simulink model "B4_quadcopter_model_discrete"  (R2021b)
settings: Solver=VariableStepAuto  StartTime=0.0  StopTime=10  FixedStep=0.002  RelTol=1e-3
values from neighbouring files (symbols this model uses):
  coef_sim_1 = tf_des_d.Denominator{1}(2)    [A11_setup_script_pprz.m]    (also in A1_setup_script.m; A6_slow_actuator.m)
  coef_sim_2 = tf_des_d.Numerator{1}(2)    [A11_setup_script_pprz.m]    (also in A1_setup_script.m; A6_slow_actuator.m)
  doublet_mag = - 0.15    (= -0.15)    [A11_setup_script_pprz.m]    (also in A1_setup_script.m)
  doublet_time = 6    [A11_setup_script_pprz.m]    (also in A1_setup_script.m)
  f_8 = 1    [A11_setup_script_pprz.m]    (also in A1_setup_script.m)
  FILT_CUTOFF = 2*pi*5    (= 31.4159265359)    [A11_setup_script_pprz.m]    (also in A1_setup_script.m)
  FILTER = 1    [A11_setup_script_pprz.m]    (also in A1_setup_script.m)
  G1 = inv(I)*G1_r    [A10_simple_plant.m]    (also in A11_setup_script_pprz.m = G1/scale; A1_setup_script.m = [G1;G1_T])
  G1_simple = inv(I)*G1_r_simple    [A1_setup_script.m]
  G2 = G2/scale    [A11_setup_script_pprz.m]    (also in A1_setup_script.m = (1/sampling_time)*inv(I)*(G2_r))
  h_plate = 0.3    [A11_setup_script_pprz.m]    (also in A1_setup_script.m = 0.16)
  I = eye(3,3)    [A10_simple_plant.m]    (also in A11_setup_script_pprz.m; A1_setup_script.m; A2_B_matrix_generation_symbolic.m = [Ixx 0 0; A3_B_matrix_generation_symbolic_cascaded.m = [Ixx 0 0)
  Iyy = 0.0008    [A11_setup_script_pprz.m]    (also in A1_setup_script.m = 0.0015)
  Izz = 0.000498    [A11_setup_script_pprz.m]    (also in A1_setup_script.m = 0.00015)
  K = 7    [A11_setup_script_pprz.m]    (also in A1_setup_script.m = 10)
  K_act = 50    [A10_simple_plant.m]    (also in A11_setup_script_pprz.m = 20; A1_setup_script.m = 20)
  K_act_outer = diag([K K K_act])    [A1_setup_script.m]
  K_d = 15    [A11_setup_script_pprz.m]    (also in A1_setup_script.m = 25)
  K_dd = K_act    (= 20)    [A11_setup_script_pprz.m]    (also in A1_setup_script.m)
  K_dyn = K    (= 10)    [A1_setup_script.m]
  K_ec = 50    [A11_setup_script_pprz.m]    (also in A1_setup_script.m = 251)
  K_ec_d = 13    [A11_setup_script_pprz.m]    (also in A1_setup_script.m = 25)
  K_ec_d_u = 1.5    [A11_setup_script_pprz.m]    (also in A1_setup_script.m = 5)
  K_ec_d_v = 1.5    [A11_setup_script_pprz.m]    (also in A1_setup_script.m = 5)
  K_ec_d_w = 1.5    [A11_setup_script_pprz.m]    (also in A1_setup_script.m = 5)
  K_ec_dd = 9    [A11_setup_script_pprz.m]    (also in A1_setup_script.m = 45)
  K_ec_i = 0    [A11_setup_script_pprz.m]    (also in A1_setup_script.m = 380)
  K_ec_u = 1.5    [A11_setup_script_pprz.m]    (also in A1_setup_script.m = 5)
  K_ec_v = 1.5    [A11_setup_script_pprz.m]    (also in A1_setup_script.m = 5)
  K_ec_w = 1.5    [A11_setup_script_pprz.m]    (also in A1_setup_script.m = 5)
  K_t = 0.0005    [A10_simple_plant.m]    (also in A11_setup_script_pprz.m = 6.557e-08; A1_setup_script.m = 6.557e-08)
  K_u = 1.0    (= 1)    [A11_setup_script_pprz.m]    (also in A1_setup_script.m = 1.5)
  K_u_d = 2.5    [A11_setup_script_pprz.m]    (also in A1_setup_script.m = 7)
  K_u_dd = K    (= 10)    [A1_setup_script.m]
  K_v = 1.0    (= 1)    [A11_setup_script_pprz.m]    (also in A1_setup_script.m = 1.5)
  K_v_d = 2.5    [A11_setup_script_pprz.m]    (also in A1_setup_script.m = 7)
  K_v_dd = K    (= 10)    [A1_setup_script.m]
  K_w = 1.0    (= 1)    [A11_setup_script_pprz.m]    (also in A1_setup_script.m = 4.5)
  K_w_d = 2.5    [A11_setup_script_pprz.m]    (also in A1_setup_script.m = 7)
  K_w_dd = K    (= 10)    [A1_setup_script.m]
  l_plate = 0.1    [A11_setup_script_pprz.m]    (also in A1_setup_script.m = 0.11)
  m = 0.4    [A10_simple_plant.m]    (also in A11_setup_script_pprz.m; A1_setup_script.m)
  NOISE = 0    [A11_setup_script_pprz.m]    (also in A1_setup_script.m)
  NOISE_ACC = 0.00005    (= 5e-05)    [A11_setup_script_pprz.m]    (also in A1_setup_script.m)
  NOISE_GYRO = 0.00005    (= 5e-05)    [A11_setup_script_pprz.m]    (also in A1_setup_script.m)
  NOISE_RPM = 200    [A11_setup_script_pprz.m]    (also in A1_setup_script.m)
  omega_act = 50    [A6_slow_actuator.m]
  omega_des = 20.00    (= 20)    [A11_setup_script_pprz.m]    (also in A1_setup_script.m; A6_slow_actuator.m = 49)
  sampling_time = 1/frequency    (= 0.002)    [A11_setup_script_pprz.m]    (also in A12_sim_multi_run.m; A1_setup_script.m; A6_slow_actuator.m)
  scale_8 = 1.6    [A11_setup_script_pprz.m]    (also in A1_setup_script.m)
  start_8 = 2    [A11_setup_script_pprz.m]    (also in A1_setup_script.m)
  start_time = 2    [A11_setup_script_pprz.m]    (also in A1_setup_script.m = 1)
  t_8 = 10    [A11_setup_script_pprz.m]    (also in A1_setup_script.m)
  w_plate = 0.3    [A11_setup_script_pprz.m]    (also in A1_setup_script.m = 0.36)
undefined symbols (not defined in the file or in its folder): DiscIntNeverNeededParam, K_ec_d_p, K_ec_d_q, K_ec_d_r, K_ec_dd_p, K_ec_dd_q, K_ec_dd_r, K_ec_i_u, K_ec_i_v, K_ec_i_w, K_ec_p, K_ec_q, K_ec_r, K_p, K_p_d, K_p_dd, K_q, K_q_d, K_q_dd, K_r, K_r_d, K_r_dd
libraries: simulink x44, cstblocks x37, dspinverses x26, dspmathops x9, dspstat3 x9, aerolibutil x9, sharedutil x3, aerolibanim x1
(part 2 of 13)

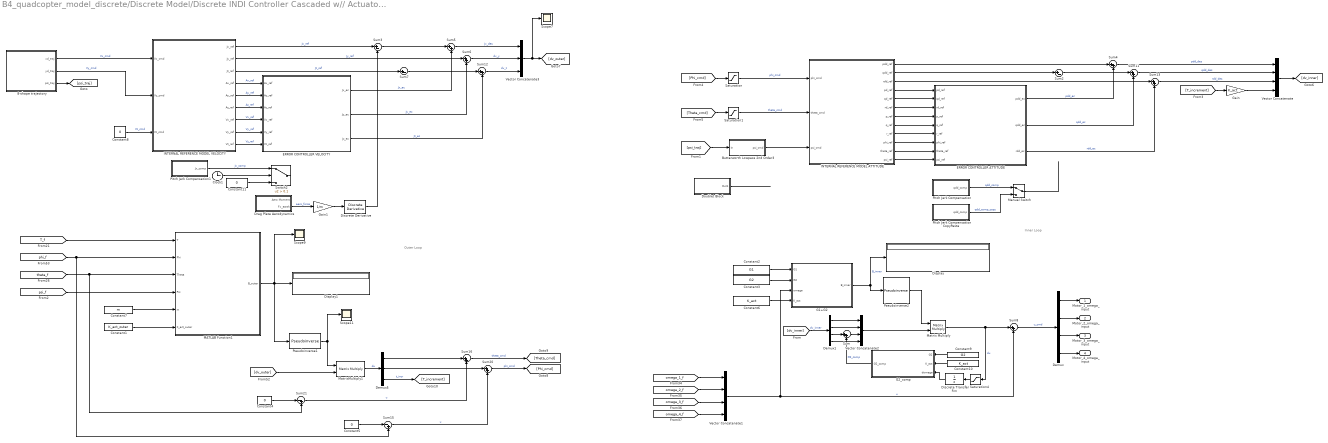
== system B4_quadcopter_model_discrete/Discrete Model/Discrete INDI Controller Cascaded w// Actuator Compensation Double ==
  note: Outer Loop
  note: Inner Loop
  8-shape trajectory : Subsystem
  Butterworth Lowpass 2nd Order3 : Subsystem
  Clock1 : Clock
      settings: Decimation=100
  Constant1 : Constant  Value=K_act_outer  SampleTime=sampling_time
  Constant10 : Constant  Value=K_act  SampleTime=sampling_time
  Constant11 : Constant  Value=0
  Constant2 : Constant  Value=G1  SampleTime=sampling_time
  Constant3 : Constant  Value=G2  SampleTime=sampling_time
  Constant4 : Constant  Value=0
  Constant5 : Constant  Value=0
  Constant6 : Constant  Value=K_act  SampleTime=sampling_time
  Constant7 : Constant  Value=m  SampleTime=sampling_time
  Constant8 : Constant  Value=0  SampleTime=sampling_time
  Constant9 : Constant  Value=G2  SampleTime=sampling_time
  Demux : Demux
  Demux1 : Demux
  Demux5 : Demux  Outputs=3
  Discrete Transfer Fcn : DiscreteTransferFcn  Denominator=[1 0]
  Discrete Derivative : simulink/Discrete/Discrete Derivative  gainval=1.0  ICPrevScaledInput=0.0  OutMin=[]  OutMax=[]  OutDataType=fixdt(1, 16)  OutScaling=2^-10  DoSatur=off
  Display : Display
  Display1 : Display
  Doublet Block : Subsystem
  Drag Plate Aerodynamics : Subsystem
  ERROR CONTROLLER ATTITUDE : Subsystem
  ERROR CONTROLLER VELOCITY : Subsystem
  G1+G2 : MATLAB Function  TreatAsAtomicUnit=on
  G2_comp : MATLAB Function  TreatAsAtomicUnit=on
  Gain : Gain  Gain=K_act
  Gain1 : Gain  Gain=1/m
  INTERNAL REFERENCE MODEL ATTITUDE : Subsystem
  INTERNAL REFERENCE MODEL VELOCITY : Subsystem
  MATLAB Function1 : MATLAB Function  TreatAsAtomicUnit=on
  Manual Switch : ManualSwitch
  Matrix Multiply : Product  Multiplication=Matrix(*)
  MatrixMultiply1 : Product  Multiplication=Matrix(*)
  Pitch Jerk Compensation : Subsystem
  Pitch Jerk Compensation CopyPaste : Subsystem
  Pitch Jerk Compensation1 : Subsystem
  Pseudoinverse1 : dspinverses/Pseudoinverse  wanterr=off  SimulateUsing=Interpreted execution
      settings: SourceProductBaseCode=DS
  Pseudoinverse2 : dspinverses/Pseudoinverse  wanterr=off  SimulateUsing=Interpreted execution
      settings: SourceProductBaseCode=DS
  Saturation : Saturate
  Saturation1 : Saturate
  Saturation4 : Saturate  UpperLimit=12000  LowerLimit=10
  Scope11 : Scope
  Scope7 : Scope
  Scope9 : Scope
  Sum{,4..6,8,11..13,16,20} (10 alike) : Sum  Inputs=|++
  Sum15 : Sum  Inputs=|-+
  Sum2 : Sum  Inputs=|+-
  Sum21 : Sum  Inputs=|-+
  Sum3 : Sum  Inputs=|+-
  Sum7 : Sum  Inputs=|+-
  Switch2 : Switch  Criteria=u2 > Threshold  Threshold=0.1
  Vector Concatenate : Concatenate  NumInputs=4
  Vector Concatenate1 : Concatenate  NumInputs=4
  Vector Concatenate2 : Concatenate  NumInputs=4
  Vector Concatenate3 : Concatenate  NumInputs=3
  Motor_1_omega_input : Outport
  Motor_2_omega_input : Outport  Port=2
  Motor_3_omega_input : Outport  Port=3
  Motor_4_omega_input : Outport  Port=4
  wires:
  Constant4/1 -> Sum21/1
  Sum16/1 -> [Theta_cmd]  "theta_cmd"
  Sum12/1 -> Vector Concatenate3/3  "dv_z"
  INTERNAL REFERENCE MODEL VELOCITY/2(Jy_ref) -> Sum6/1  "Jy_ref"
  Sum21/1 -> Sum16/2  "u"
  ERROR CONTROLLER VELOCITY/2(Jy_ec) -> Sum6/2  "Jy_ec"
  8-shape trajectory/1(xd_traj) -> INTERNAL REFERENCE MODEL VELOCITY/1(Vx_cmd)  "Vx_cmd"
  Sum6/1 -> Vector Concatenate3/2  "dv_y"
  ERROR CONTROLLER VELOCITY/1(Jx_ec) -> Sum5/2  "Jx_ec"
  Sum5/1 -> Vector Concatenate3/1  "Jx_des"
  ERROR CONTROLLER VELOCITY/3(Jz_ec) -> Sum12/2  "Jz_ec"
  Constant8/1 -> INTERNAL REFERENCE MODEL VELOCITY/3(Vz_cmd)  "Vz_cmd"
  Pseudoinverse1/1 -> Scope11/1, MatrixMultiply1/1
  Sum15/1 -> Sum20/2  "u"
  Vector Concatenate3/1 -> Scope7/1, [dv_outer]
  INTERNAL REFERENCE MODEL VELOCITY/1(Jx_ref) -> Sum3/1  "Jx_ref"
  INTERNAL REFERENCE MODEL VELOCITY/3(Jz_ref) -> Sum7/1  "Jz_ref"
  Sum20/1 -> [Phi_cmd]  "phi_cmd"
  [T_f] -> MATLAB Function1/1(T)
  Constant7/1 -> MATLAB Function1/5(m)
  Constant5/1 -> Sum15/1
  [dv_outer] -> MatrixMultiply1/2
  Demux5/1 -> Sum16/1
  MATLAB Function1/1(B_outer) -> Pseudoinverse1/1, Display1/1, Scope9/1
  Demux5/3 -> [T_increment]  "t_incr"
  MatrixMultiply1/1 -> Demux5/1  "du"
  Demux5/2 -> Sum20/1
  8-shape trajectory/2(yd_traj) -> INTERNAL REFERENCE MODEL VELOCITY/2(Vy_cmd)  "Vy_cmd"
  [theta_f] -> Sum21/2, MATLAB Function1/3(Theta)
  [phi_f] -> Sum15/2, MATLAB Function1/2(Phi)
  8-shape trajectory/3(psi_traj) -> [psi_traj]
  INTERNAL REFERENCE MODEL VELOCITY/4(Ax_ref) -> ERROR CONTROLLER VELOCITY/1(Ax_ref)  "Ax_ref"
  INTERNAL REFERENCE MODEL VELOCITY/5(Ay_ref) -> ERROR CONTROLLER VELOCITY/2(Ay_ref)  "Ay_ref"
  INTERNAL REFERENCE MODEL VELOCITY/6(Az_ref) -> ERROR CONTROLLER VELOCITY/3(Az_ref)  "Az_ref"
  INTERNAL REFERENCE MODEL VELOCITY/7(Vx_ref) -> ERROR CONTROLLER VELOCITY/4(Vx_ref)  "Vx_ref"
  INTERNAL REFERENCE MODEL VELOCITY/8(Vy_ref) -> ERROR CONTROLLER VELOCITY/5(Vy_ref)  "Vy_ref"
  INTERNAL REFERENCE MODEL VELOCITY/9(Vz_ref) -> ERROR CONTROLLER VELOCITY/6(Vz_ref)  "Vz_ref"
  Sum3/1 -> Sum5/1
  Sum7/1 -> Sum12/1
  Constant1/1 -> MATLAB Function1/6(K_act_outer)
  [psi_f] -> MATLAB Function1/4(Psi)
  INTERNAL REFERENCE MODEL ATTITUDE/12(psi_ref) -> ERROR CONTROLLER ATTITUDE/9(psi_ref)
  Demux1/1 -> Vector Concatenate2/1
  ERROR CONTROLLER ATTITUDE/2(qdd_ec) -> Sum11/2  "qdd_ec"
  Sum4/1 -> Vector Concatenate/1  "pdd_des"
  [dv_inner] -> Demux1/1  "dv_inner"
  Demux1/4 -> Vector Concatenate2/4
  INTERNAL REFERENCE MODEL ATTITUDE/3(rdd_ref) -> Sum13/1
  Sum2/1 -> Sum11/1
  INTERNAL REFERENCE MODEL ATTITUDE/9(r_ref) -> ERROR CONTROLLER ATTITUDE/6(r_ref)
  [omega_2_f] -> Vector Concatenate1/2
  Sum11/1 -> Vector Concatenate/2  "qdd_des"
  INTERNAL REFERENCE MODEL ATTITUDE/10(phi_ref) -> ERROR CONTROLLER ATTITUDE/7(phi_ref)
  Demux1/2 -> Vector Concatenate2/2
  G2_comp/1(G2_comp) -> Sum/2  "G2_comp"
  Saturation1/1 -> INTERNAL REFERENCE MODEL ATTITUDE/2(theta_cmd)  "theta_cmd"
  [Theta_cmd] -> Saturation1/1
  Demux/3 -> Motor_3_omega_input/1
  INTERNAL REFERENCE MODEL ATTITUDE/4(pd_ref) -> ERROR CONTROLLER ATTITUDE/1(pd_ref)
  Saturation/1 -> INTERNAL REFERENCE MODEL ATTITUDE/1(phi_cmd)  "phi_cmd"
  Doublet Block/1(Out1) -> ?
  INTERNAL REFERENCE MODEL ATTITUDE/7(p_ref) -> ERROR CONTROLLER ATTITUDE/4(p_ref)
  Sum/1 -> Vector Concatenate2/3
  Demux1/3 -> Sum/1
  [omega_1_f] -> Vector Concatenate1/1
  INTERNAL REFERENCE MODEL ATTITUDE/2(qdd_ref) -> Sum2/1
  INTERNAL REFERENCE MODEL ATTITUDE/11(theta_ref) -> ERROR CONTROLLER ATTITUDE/8(theta_ref)
  Constant3/1 -> G1+G2/2(G2)
  Vector Concatenate1/1 -> G1+G2/3(omega), Sum8/2  "u"
  Saturation4/1 -> Discrete Transfer Fcn/1
  Pseudoinverse2/1 -> Matrix Multiply/1
  Demux/4 -> Motor_4_omega_input/1
  Butterworth Lowpass 2nd Order3/1(psi_cmd) -> INTERNAL REFERENCE MODEL ATTITUDE/3(psi_cmd)
  Sum13/1 -> Vector Concatenate/3  "rdd_des"
  Vector Concatenate2/1 -> Matrix Multiply/2
  ERROR CONTROLLER ATTITUDE/3(rdd_ec) -> Sum13/2  "rdd_ec"
  Constant10/1 -> G2_comp/2(K_act)
  [omega_4_f] -> Vector Concatenate1/4
  ERROR CONTROLLER ATTITUDE/1(pdd_ec) -> Sum4/2  "pdd_ec"
  Discrete Transfer Fcn/1 -> G2_comp/3(domega)
  INTERNAL REFERENCE MODEL ATTITUDE/8(q_ref) -> ERROR CONTROLLER ATTITUDE/5(q_ref)
  Pitch Jerk Compensation CopyPaste/1(qdd_comp) -> Manual Switch/2  "qdd_comp_copy"
  Demux/2 -> Motor_2_omega_input/1
  Constant2/1 -> G1+G2/1(G1)
  Constant9/1 -> G2_comp/1(G2)
  INTERNAL REFERENCE MODEL ATTITUDE/1(pdd_ref) -> Sum4/1
  G1+G2/1(B_inner) -> Pseudoinverse2/1, Display/1  "B_inner"
  [T_increment] -> Gain/1
  Demux/1 -> Motor_1_omega_input/1
  [psi_traj] -> Butterworth Lowpass 2nd Order3/1(In)
  Constant6/1 -> G1+G2/4(K_act)
  INTERNAL REFERENCE MODEL ATTITUDE/6(rd_ref) -> ERROR CONTROLLER ATTITUDE/3(rd_ref)
  Manual Switch/1 -> ?
  Vector Concatenate/1 -> [dv_inner]
  Sum8/1 -> Demux/1  "u_cmd"
  [omega_3_f] -> Vector Concatenate1/3
  INTERNAL REFERENCE MODEL ATTITUDE/5(qd_ref) -> ERROR CONTROLLER ATTITUDE/2(qd_ref)
  Gain/1 -> Vector Concatenate/4
  [Phi_cmd] -> Saturation/1
  Matrix Multiply/1 -> Saturation4/1, Sum8/1  "du"
  Pitch Jerk Compensation/1(qdd_comp) -> Manual Switch/1  "qdd_comp"
  Constant11/1 -> Switch2/3
  Pitch Jerk Compensation1/1(Jx_comp) -> Switch2/1  "Jx_comp"
  Clock1/1 -> Switch2/2
  Drag Plate Aerodynamics/2(Fx_earth) -> Gain1/1  "aero_force"
  Gain1/1 -> Discrete Derivative/1
  Discrete Derivative/1 -> Sum3/2

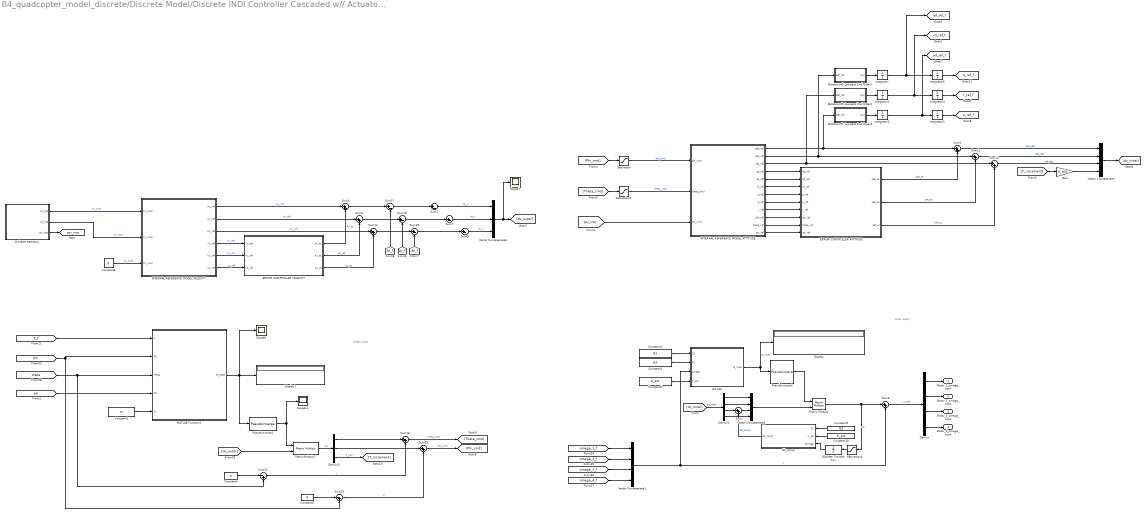
== system B4_quadcopter_model_discrete/Discrete Model/Discrete INDI Controller Cascaded w// Actuator Compensation1 ==
  note: Inner Loop
  note: Outer Loop
  8-shape trajectory : Subsystem
  Butterworth Lowpass 2nd Order1 : Subsystem
  Butterworth Lowpass 2nd Order2 : Subsystem
  Butterworth Lowpass 2nd Order3 : Subsystem
  Constant1 : Constant  Value=m  SampleTime=sampling_time
  Constant10 : Constant  Value=K_act  SampleTime=sampling_time
  Constant2 : Constant  Value=G1  SampleTime=sampling_time
  Constant3 : Constant  Value=G2  SampleTime=sampling_time
  Constant4 : Constant  Value=0
  Constant5 : Constant  Value=0
  Constant6 : Constant  Value=K_act  SampleTime=sampling_time
  Constant8 : Constant  Value=0  SampleTime=sampling_time
  Constant9 : Constant  Value=G2  SampleTime=sampling_time
  Demux : Demux
  Demux1 : Demux
  Demux5 : Demux  Outputs=3
  Discrete Transfer Fcn : DiscreteTransferFcn  Denominator=[1 0]
  Display : Display
  Display1 : Display
  ERROR CONTROLLER ATTITUDE : Subsystem
  ERROR CONTROLLER VELOCITY : Subsystem
  G1+G2 : MATLAB Function  TreatAsAtomicUnit=on
  G2_comp : MATLAB Function  TreatAsAtomicUnit=on
  Gain : Gain  Gain=K_act
  INTERNAL REFERENCE MODEL ATTITUDE : Subsystem
  INTERNAL REFERENCE MODEL VELOCITY : Subsystem
  Integrator{,1..5} (6 alike) : Integrator
  MATLAB Function1 : MATLAB Function  TreatAsAtomicUnit=on
  Matrix Multiply : Product  Multiplication=Matrix(*)
  MatrixMultiply1 : Product  Multiplication=Matrix(*)
  Pseudoinverse1 : dspinverses/Pseudoinverse  wanterr=off  SimulateUsing=Interpreted execution
      settings: SourceProductBaseCode=DS
  Pseudoinverse2 : dspinverses/Pseudoinverse  wanterr=off  SimulateUsing=Interpreted execution
      settings: SourceProductBaseCode=DS
  Saturation : Saturate
  Saturation1 : Saturate
  Saturation4 : Saturate  UpperLimit=12000  LowerLimit=10
  Scope11 : Scope
  Scope7 : Scope
  Scope9 : Scope
  Sum{,4..6,8,11..13,16,20} (10 alike) : Sum  Inputs=|++
  Sum15 : Sum  Inputs=|-+
  Sum{3,7,9,17..19} (6 alike) : Sum  Inputs=|+-
  Sum21 : Sum  Inputs=|-+
  Vector Concatenate : Concatenate  NumInputs=4
  Vector Concatenate1 : Concatenate  NumInputs=4
  Vector Concatenate2 : Concatenate  NumInputs=4
  Vector Concatenate3 : Concatenate  NumInputs=3
  Motor_1_omega_input : Outport
  Motor_2_omega_input : Outport  Port=2
  Motor_3_omega_input : Outport  Port=3
  Motor_4_omega_input : Outport  Port=4
  tag scope: p_ref_f=global, pd_ref_f=global, psi_traj=global, q_ref_f=global, qd_ref_f=global, r_ref_f=global, rd_ref_f=global
  wires:
  G1+G2/1(B_inner) -> Pseudoinverse2/1, Display/1  "B_inner"
  Vector Concatenate1/1 -> G1+G2/3(omega), Sum8/2  "u"
  Vector Concatenate/1 -> [dv_inner]
  Matrix Multiply/1 -> Saturation4/1, Sum8/1  "du"
  Demux/1 -> Motor_1_omega_input/1
  [omega_4_f] -> Vector Concatenate1/4
  [omega_2_f] -> Vector Concatenate1/2
  Demux/3 -> Motor_3_omega_input/1
  Sum8/1 -> Demux/1  "u_cmd"
  Pseudoinverse2/1 -> Matrix Multiply/1
  [omega_1_f] -> Vector Concatenate1/1
  Demux/2 -> Motor_2_omega_input/1
  Demux/4 -> Motor_4_omega_input/1
  [omega_3_f] -> Vector Concatenate1/3
  INTERNAL REFERENCE MODEL VELOCITY/5(Vy_ref) -> ERROR CONTROLLER VELOCITY/2(Vy_ref)  "Vy_ref"
  Constant4/1 -> Sum21/1
  Sum16/1 -> [Theta_cmd]  "theta_cmd"
  Sum9/1 -> Vector Concatenate3/3  "dv_z"
  INTERNAL REFERENCE MODEL VELOCITY/2(Ay_ref) -> Sum6/1  "Ay_ref"
  Sum21/1 -> Sum16/2  "u"
  INTERNAL REFERENCE MODEL VELOCITY/6(Vz_ref) -> ERROR CONTROLLER VELOCITY/3(Vz_ref)  "Vz_ref"
  INTERNAL REFERENCE MODEL VELOCITY/4(Vx_ref) -> ERROR CONTROLLER VELOCITY/1(Vx_ref)  "Vx_ref"
  ERROR CONTROLLER VELOCITY/2(Ay_ec) -> Sum6/2  "Ay_ec"
  8-shape trajectory/1(xd_traj) -> INTERNAL REFERENCE MODEL VELOCITY/1(Vx_cmd)  "Vx_cmd"
  Sum7/1 -> Vector Concatenate3/2  "dv_y"
  ERROR CONTROLLER VELOCITY/1(Ax_ec) -> Sum5/2  "Ax_ec"
  Sum3/1 -> Vector Concatenate3/1  "dv_x"
  ERROR CONTROLLER VELOCITY/3(Az_ec) -> Sum12/2  "Az_ec"
  Sum12/1 -> Sum19/1
  Constant8/1 -> INTERNAL REFERENCE MODEL VELOCITY/3(Vz_cmd)  "Vz_cmd"
  Pseudoinverse1/1 -> Scope11/1, MatrixMultiply1/1
  Sum15/1 -> Sum20/2  "u"
  Vector Concatenate3/1 -> Scope7/1, [dv_outer]
  INTERNAL REFERENCE MODEL VELOCITY/1(Ax_ref) -> Sum5/1  "Ax_ref"
  INTERNAL REFERENCE MODEL VELOCITY/3(Az_ref) -> Sum12/1  "Az_ref"
  Sum20/1 -> [Phi_cmd]  "phi_cmd"
  [T_f] -> MATLAB Function1/1(T)
  Sum6/1 -> Sum18/1
  Constant5/1 -> Sum15/1
  [dv_outer] -> MatrixMultiply1/2
  MATLAB Function1/1(B_outer) -> Scope9/1, Display1/1, Pseudoinverse1/1
  Demux5/3 -> [T_increment]  "t_incr"
  MatrixMultiply1/1 -> Demux5/1  "du"
  8-shape trajectory/2(yd_traj) -> INTERNAL REFERENCE MODEL VELOCITY/2(Vy_cmd)  "Vy_cmd"
  [T_increment] -> Gain/1
  [Ax_f] -> Sum17/2
  [Ay_f] -> Sum18/2
  [Az_f] -> Sum19/2
  [Phi_cmd] -> Saturation/1
  [theta] -> Sum21/2, MATLAB Function1/3(Theta)
  [phi] -> Sum15/2, MATLAB Function1/2(Phi)
  INTERNAL REFERENCE MODEL ATTITUDE/4(pd_ref) -> ERROR CONTROLLER ATTITUDE/1(pd_ref)
  INTERNAL REFERENCE MODEL ATTITUDE/7(p_ref) -> ERROR CONTROLLER ATTITUDE/4(p_ref)
  ERROR CONTROLLER ATTITUDE/3(rdd_ec) -> Sum13/2  "rdd_ec"
  ERROR CONTROLLER ATTITUDE/2(qdd_ec) -> Sum11/2  "qdd_ec"
  INTERNAL REFERENCE MODEL ATTITUDE/5(qd_ref) -> ERROR CONTROLLER ATTITUDE/2(qd_ref)
  INTERNAL REFERENCE MODEL ATTITUDE/11(theta_ref) -> ERROR CONTROLLER ATTITUDE/8(theta_ref)
  INTERNAL REFERENCE MODEL ATTITUDE/1(pdd_ref) -> Sum4/1, Butterworth Lowpass 2nd Order3/1(qdd_ref)
  INTERNAL REFERENCE MODEL ATTITUDE/3(rdd_ref) -> Butterworth Lowpass 2nd Order2/1(qdd_ref), Sum13/1
  INTERNAL REFERENCE MODEL ATTITUDE/8(q_ref) -> ERROR CONTROLLER ATTITUDE/5(q_ref)
  ERROR CONTROLLER ATTITUDE/1(pdd_ec) -> Sum4/2  "pdd_ec"
  INTERNAL REFERENCE MODEL ATTITUDE/6(rd_ref) -> ERROR CONTROLLER ATTITUDE/3(rd_ref)
  INTERNAL REFERENCE MODEL ATTITUDE/10(phi_ref) -> ERROR CONTROLLER ATTITUDE/7(phi_ref)
  INTERNAL REFERENCE MODEL ATTITUDE/12(psi_ref) -> ERROR CONTROLLER ATTITUDE/9(psi_ref)
  INTERNAL REFERENCE MODEL ATTITUDE/9(r_ref) -> ERROR CONTROLLER ATTITUDE/6(r_ref)
  Sum13/1 -> Vector Concatenate/3  "rdd_des"
  Sum4/1 -> Vector Concatenate/1  "pdd_des"
  Sum11/1 -> Vector Concatenate/2  "qdd_des"
  Gain/1 -> Vector Concatenate/4
  Constant3/1 -> G1+G2/2(G2)
  Constant6/1 -> G1+G2/4(K_act)
  Constant2/1 -> G1+G2/1(G1)
  Constant9/1 -> G2_comp/1(G2)
  Constant10/1 -> G2_comp/2(K_act)
  Discrete Transfer Fcn/1 -> G2_comp/3(domega)
  [dv_inner] -> Demux1/1  "dv_inner"
  Sum/1 -> Vector Concatenate2/3
  Demux1/3 -> Sum/1
  Demux1/2 -> Vector Concatenate2/2
  Demux1/1 -> Vector Concatenate2/1
  Demux1/4 -> Vector Concatenate2/4
  Vector Concatenate2/1 -> Matrix Multiply/2
  G2_comp/1(G2_comp) -> Sum/2  "G2_comp"
  Sum5/1 -> Sum17/1
  INTERNAL REFERENCE MODEL ATTITUDE/2(qdd_ref) -> Butterworth Lowpass 2nd Order1/1(qdd_ref), Sum11/1
  8-shape trajectory/3(psi_traj) -> [psi_traj]
  [Theta_cmd] -> Saturation1/1
  Saturation4/1 -> Discrete Transfer Fcn/1
  Saturation/1 -> INTERNAL REFERENCE MODEL ATTITUDE/1(phi_cmd)  "phi_cmd"
  Sum17/1 -> Sum3/1
  Sum18/1 -> Sum7/1
  Sum19/1 -> Sum9/1
  Constant1/1 -> MATLAB Function1/5(m)
  Demux5/2 -> Sum20/1
  Demux5/1 -> Sum16/1
  [psi] -> MATLAB Function1/4(Psi)
  Saturation1/1 -> INTERNAL REFERENCE MODEL ATTITUDE/2(theta_cmd)  "theta_cmd"
  [psi_traj] -> INTERNAL REFERENCE MODEL ATTITUDE/3(psi_cmd)
  Butterworth Lowpass 2nd Order1/1(Out) -> Integrator/1
  Integrator/1 -> [qd_ref_f], Integrator5/1
  Integrator1/1 -> Integrator4/1, [rd_ref_f]
  Butterworth Lowpass 2nd Order2/1(Out) -> Integrator1/1
  Integrator2/1 -> Integrator3/1, [pd_ref_f]
  Butterworth Lowpass 2nd Order3/1(Out) -> Integrator2/1
  Integrator3/1 -> [p_ref_f]
  Integrator4/1 -> [r_ref_f]
  Integrator5/1 -> [q_ref_f]

== system B4_quadcopter_model_discrete/Discrete Model/Force and Moment Calculation ==
  omega_1 : Inport
  omega_2 : Inport  Port=2
  omega_3 : Inport  Port=3
  omega_4 : Inport  Port=4
  Add : Sum
  Add1 : Sum
  Constant : Constant  Value=0
  Constant1 : Constant  Value=sampling_time  SampleTime=sampling_time
  Constant2 : Constant  Value=G1  SampleTime=sampling_time
  Constant3 : Constant  Value=G2  SampleTime=sampling_time
  Constant4 : Constant  Value=K_t  SampleTime=sampling_time
  Constant5 : Constant  Value=I  SampleTime=sampling_time
  Derivative : Derivative
  Drag Plate Aerodynamics : Subsystem
  Forces due to thrust : MATLAB Function  TreatAsAtomicUnit=on
  Gain : Gain  Gain=0.09
  Gain1 : Gain  Gain=0.09
  Moments due to thrust : MATLAB Function  TreatAsAtomicUnit=on
  Mux : Mux
  Mux1 : Mux  Inputs=3
  Sum : Sum  Inputs=|++
  Moments in body frame : Outport
  Forces in earth frame : Outport  Port=2
  Collective Thrust : Outport  Port=3
  wires:
  Moments due to thrust/1(M_t) -> Add1/2  "thrust_moment"
  Constant2/1 -> Moments due to thrust/3(G1)
  Constant3/1 -> Moments due to thrust/4(G2)
  omega_4/1 -> Forces due to thrust/4(omega_4), Mux/4
  omega_3/1 -> Forces due to thrust/3(omega_3), Mux/3
  omega_2/1 -> Forces due to thrust/2(omega_2), Mux/2
  omega_1/1 -> Forces due to thrust/1(omega_1), Mux/1
  Mux/1 -> Derivative/1, Moments due to thrust/1(omega)
  Derivative/1 -> Moments due to thrust/2(omega_dot)
  Constant1/1 -> Moments due to thrust/5(sampling_time)
  [R_bg] -> Forces due to thrust/5(R_bg)
  Constant4/1 -> Forces due to thrust/6(K_t)
  Forces due to thrust/1(F_t_e) -> Add/2  "thrust_earth"
  Forces due to thrust/2(F_t_b) -> Collective Thrust/1  "thrust_body"
  Add/1 -> Forces in earth frame/1  "total_force"
  Add1/1 -> Moments in body frame/1  "total_moment"
  Constant5/1 -> Moments due to thrust/6(I)
  Drag Plate Aerodynamics/2(Aero Force) -> ?  "aero_force"
  Drag Plate Aerodynamics/1(Aero Moment) -> ?  "aero_moment"
  Constant/1 -> Mux1/3, Mux1/1
  [theta_cont] -> Gain/1
  [phi_cont] -> Gain1/1
  Gain/1 -> Sum/1
  Gain1/1 -> Sum/2
  Sum/1 -> Mux1/2
  Mux1/1 -> ?  "dummy_moment"

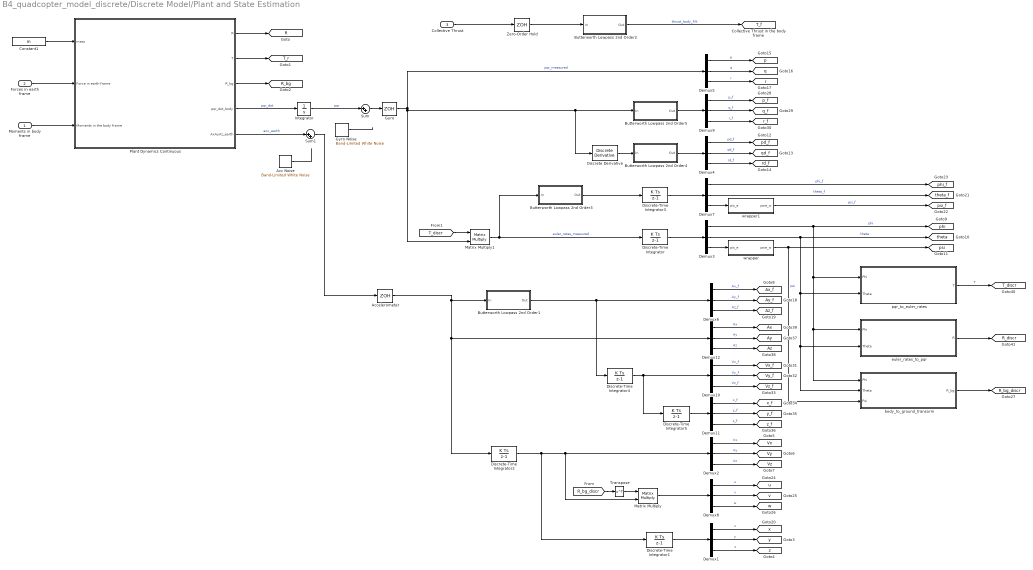
== system B4_quadcopter_model_discrete/Discrete Model/Plant and State Estimation ==
  Moments in body frame : Inport
  Forces in earth frame : Inport  Port=2
  Collective Thrust : Inport  Port=3
  Acc Noise : simulink/Sources/Band-Limited White Noise  Cov=[NOISE_ACC]  Ts=sampling_time  seed=[23341]
  Accelerometer : ZeroOrderHold  SampleTime=sampling_time
  Butterworth Lowpass 2nd Order1 : Subsystem
  Butterworth Lowpass 2nd Order2 : Subsystem
  Butterworth Lowpass 2nd Order3 : Subsystem
  Butterworth Lowpass 2nd Order4 : Subsystem
  Butterworth Lowpass 2nd Order5 : Subsystem
  Constant1 : Constant  Value=m  SampleTime=sampling_time
  Demux{1..12} (12 alike) : Demux  Outputs=3
  Discrete Derivative : simulink/Discrete/Discrete Derivative  gainval=1.0  ICPrevScaledInput=0.0  OutMin=[]  OutMax=[]  OutDataType=fixdt(1, 16)  OutScaling=2^-10  DoSatur=off
  Discrete-Time Integrator{,1..5} (6 alike) : DiscreteIntegrator  SampleTime=sampling_time  ICPrevOutput=DiscIntNeverNeededParam  ICPrevScaledInput=DiscIntNeverNeededParam
  Gyro : ZeroOrderHold  SampleTime=sampling_time
  Gyro Noise : simulink/Sources/Band-Limited White Noise  Cov=[NOISE_GYRO]  Ts=sampling_time  seed=[23341]
  Integrator : Integrator
  Matrix Multiply : Product  Multiplication=Matrix(*)
  Matrix Multiply1 : Product  Multiplication=Matrix(*)
  Plant Dynamics Continuous : Subsystem
  Sum : Sum  Inputs=|++
  Sum1 : Sum  Inputs=|++
  Transpose : Math  Operator=transpose  SaturateOnIntegerOverflow=on
  Zero-Order Hold : ZeroOrderHold  SampleTime=sampling_time
  body_to_ground_transorm : MATLAB Function  Description=|  TreatAsAtomicUnit=on
      | This function computes the rotational matrix to pass from the body frame to the world frame. 
      | Takes as inpout the euler angles.
  euler_rates_to_pqr : MATLAB Function  TreatAsAtomicUnit=on
  pqr_to_euler_rates : MATLAB Function  TreatAsAtomicUnit=on
  wrapper : MATLAB Function  TreatAsAtomicUnit=on
  wrapper1 : MATLAB Function  TreatAsAtomicUnit=on
  tag scope: Ax=global, Ax_f=global, Ay=global, Ay_f=global, Az=global, Az_f=global, R=global, R_bg=global, R_bg_discr=global, R_discr=global, T_discr=global, T_f=global, T_r=global, Vx=global, Vx_f=global, Vy=global, Vy_f=global, Vz=global, Vz_f=global, p=global, p_f=global, pd_f=global, phi=global, phi_f=global, psi=global, psi_f=global, q=global, q_f=global, qd_f=global, r=global, r_f=global, rd_f=global, theta=global, theta_f=global, u=global, v=global, w=global, x=global, x_f=global, y=global, y_f=global, z=global, z_f=global
  wires:
  Demux3/2 -> body_to_ground_transorm/2(Theta), euler_rates_to_pqr/2(Theta), pqr_to_euler_rates/2(Theta), [theta]  "theta"
  Demux4/1 -> [pd_f]  "pd_f"
  Demux3/1 -> body_to_ground_transorm/1(Phi), euler_rates_to_pqr/1(Phi), pqr_to_euler_rates/1(Phi), [phi]  "phi"
  Demux4/2 -> [qd_f]  "qd_f"
  Demux3/3 -> wrapper/1(pis_e)
  Discrete-Time Integrator/1 -> Demux3/1
  Demux5/2 -> [q]  "q"
  Demux5/1 -> [p]  "p"
  Plant Dynamics Continuous/4(pqr_dot_body) -> Integrator/1  "pqr_dot"
  Demux5/3 -> [r]  "r"
  Integrator/1 -> Sum/1  "pqr"
  Discrete Derivative/1 -> Butterworth Lowpass 2nd Order4/1(In)
  Demux4/3 -> [rd_f]  "rd_f"
  Moments in body frame/1 -> Plant Dynamics Continuous/3(Moments in the body frame)
  Constant1/1 -> Plant Dynamics Continuous/1(mass)
  Forces in earth frame/1 -> Plant Dynamics Continuous/2(Force in earth frame)
  Plant Dynamics Continuous/1(R) -> [R]
  Plant Dynamics Continuous/2(T) -> [T_r]
  Plant Dynamics Continuous/3(R_bg) -> [R_bg]
  Demux2/2 -> [Vy]  "Vy"
  Demux6/2 -> [Ay_f]  "Ay_f"
  Discrete-Time Integrator1/1 -> Demux1/1
  Demux6/1 -> [Ax_f]  "Ax_f"
  Accelerometer/1 -> Discrete-Time Integrator2/1, Demux12/1, Butterworth Lowpass 2nd Order1/1(In)
  Demux2/1 -> [Vx]  "Vx"
  Demux1/2 -> [y]  "y"
  Demux1/1 -> [x]  "x"
  Demux1/3 -> [z]  "z"
  Demux6/3 -> [Az_f]  "Az_f"
  Discrete-Time Integrator2/1 -> Demux2/1, Matrix Multiply/2, Discrete-Time Integrator1/1
  Demux2/3 -> [Vz]  "Vz"
  Plant Dynamics Continuous/5(AxAyAz_earth) -> Sum1/1  "acc_earth"
  Demux7/3 -> wrapper1/1(pis_e)
  Demux7/1 -> [phi_f]  "phi_f"
  Demux7/2 -> [theta_f]  "theta_f"
  Discrete-Time Integrator3/1 -> Demux7/1
  [R_bg_discr] -> Transpose/1
  Transpose/1 -> Matrix Multiply/1
  Demux8/2 -> [v]  "v"
  Demux8/1 -> [u]  "u"
  Demux8/3 -> [w]  "w"
  Matrix Multiply/1 -> Demux8/1
  Gyro/1 -> Discrete Derivative/1, Butterworth Lowpass 2nd Order5/1(In), Matrix Multiply1/2, Demux5/1  "pqr_measured"
  Zero-Order Hold/1 -> Butterworth Lowpass 2nd Order2/1(In)
  Butterworth Lowpass 2nd Order2/1(Out) -> [T_f]  "thrust_body_filt"
  Collective Thrust/1 -> Zero-Order Hold/1
  Demux9/3 -> [r_f]  "r_f"
  Demux9/1 -> [p_f]  "p_f"
  Demux9/2 -> [q_f]  "q_f"
  Demux10/1 -> [Vx_f]  "Vx_f"
  Demux10/2 -> [Vy_f]  "Vy_f"
  Demux10/3 -> [Vz_f]  "Vz_f"
  Demux11/2 -> [y_f]  "y_f"
  Discrete-Time Integrator5/1 -> Demux11/1
  Demux11/1 -> [x_f]  "x_f"
  Demux11/3 -> [z_f]  "z_f"
  Discrete-Time Integrator4/1 -> Discrete-Time Integrator5/1, Demux10/1
  Demux12/2 -> [Ay]  "Ay"
  Demux12/1 -> [Ax]  "Ax"
  Demux12/3 -> [Az]  "Az"
  [T_discr] -> Matrix Multiply1/1
  Matrix Multiply1/1 -> Butterworth Lowpass 2nd Order3/1(In), Discrete-Time Integrator/1  "euler_rates_measured"
  Butterworth Lowpass 2nd Order3/1(Out) -> Discrete-Time Integrator3/1
  euler_rates_to_pqr/1(R) -> [R_discr]
  pqr_to_euler_rates/1(T) -> [T_discr]  "T"
  body_to_ground_transorm/1(R_bg) -> [R_bg_discr]
  Butterworth Lowpass 2nd Order1/1(Out) -> Demux6/1, Discrete-Time Integrator4/1
  wrapper/1(psie_w) -> body_to_ground_transorm/3(Psi), [psi]  "psi"
  wrapper1/1(psie_w) -> [psi_f]  "psi_f"
  Sum/1 -> Gyro/1
  Gyro Noise/1 -> ?
  Acc Noise/1 -> ?
  Sum1/1 -> Accelerometer/1
  Butterworth Lowpass 2nd Order5/1(Out) -> Demux9/1
  Butterworth Lowpass 2nd Order4/1(Out) -> Demux4/1

== system B4_quadcopter_model_discrete/Discrete Model - Complementary Filtering/Continuous Actuator Dynamics ==
  Motor_1_omega_input : Inport
  Motor_2_omega_input : Inport  Port=2
  Motor_3_omega_input : Inport  Port=3
  Motor_4_omega_input : Inport  Port=4
  Demux : Demux
  Discrete Transfer Fcn{1..4} (4 alike) : DiscreteTransferFcn  Numerator=[coef_sim_2]  Denominator=[1 coef_sim_1]  SampleTime=sampling_time
  Mux : Mux
  Noise RPM : Subsystem
  Saturation{,1..3} (4 alike) : Saturate  UpperLimit=12000  LowerLimit=10
  Sum : Sum  Inputs=|++
  Transfer Fcn{,1..3} (4 alike) : TransferFcn  Numerator=[omega_des]  Denominator=[1 omega_des]
  omega_1 : Outport
  omega_2 : Outport  Port=2
  omega_3 : Outport  Port=3
  omega_4 : Outport  Port=4
  tag scope: omega_1_f=global, omega_2_f=global, omega_3_f=global, omega_4_f=global
  wires:
  Transfer Fcn3/1 -> omega_4/1  "omega_4"
  Motor_4_omega_input/1 -> Saturation3/1  "omega_4_in"
  Saturation/1 -> Discrete Transfer Fcn2/1, Transfer Fcn/1
  Motor_3_omega_input/1 -> Saturation2/1  "omega_3_in"
  Transfer Fcn1/1 -> omega_2/1  "omega_2"
  Saturation1/1 -> Transfer Fcn1/1, Discrete Transfer Fcn1/1
  Saturation3/1 -> Transfer Fcn3/1, Discrete Transfer Fcn4/1
  Discrete Transfer Fcn2/1 -> Mux/1
  Saturation2/1 -> Transfer Fcn2/1, Discrete Transfer Fcn3/1
  Motor_2_omega_input/1 -> Saturation1/1  "omega_2_in"
  Demux/2 -> [omega_2_f]  "omega_2_est"
  Motor_1_omega_input/1 -> Saturation/1  "omega_1_in"
  Transfer Fcn/1 -> omega_1/1  "omega_1"
  Demux/4 -> [omega_4_f]  "omega_4_est"
  Discrete Transfer Fcn4/1 -> Mux/4
  Discrete Transfer Fcn1/1 -> Mux/2
  Discrete Transfer Fcn3/1 -> Mux/3
  Transfer Fcn2/1 -> omega_3/1  "omega_3"
  Demux/1 -> [omega_1_f]  "omega_1_est"
  Demux/3 -> [omega_3_f]  "omega_3_est"
  Sum/1 -> Demux/1
  Mux/1 -> Sum/1  "pqr_measured"
  Noise RPM/1(Out) -> Sum/2

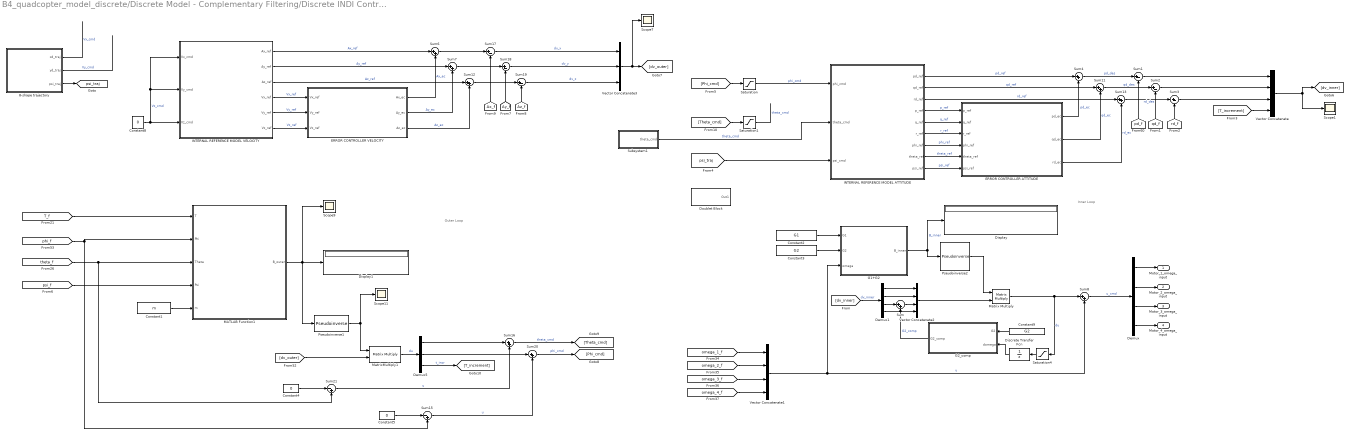
== system B4_quadcopter_model_discrete/Discrete Model - Complementary Filtering/Discrete INDI Controller Cascaded ==
  note: Inner Loop
  note: Outer Loop
  8-shape trajectory : Subsystem
  Constant1 : Constant  Value=m  SampleTime=sampling_time
  Constant2 : Constant  Value=G1  SampleTime=sampling_time
  Constant3 : Constant  Value=G2  SampleTime=sampling_time
  Constant4 : Constant  Value=0
  Constant5 : Constant  Value=0
  Constant8 : Constant  Value=0  SampleTime=sampling_time
  Constant9 : Constant  Value=G2  SampleTime=sampling_time
  Demux : Demux
  Demux1 : Demux
  Demux5 : Demux  Outputs=3
  Discrete Transfer Fcn : DiscreteTransferFcn  Denominator=[1 0]
  Display : Display
  Display1 : Display
  Doublet Block : Subsystem
  ERROR CONTROLLER ATTITUDE : Subsystem
  ERROR CONTROLLER VELOCITY : Subsystem
  G1+G2 : MATLAB Function  TreatAsAtomicUnit=on
  G2_comp : MATLAB Function  TreatAsAtomicUnit=on
  INTERNAL REFERENCE MODEL ATTITUDE : Subsystem
  INTERNAL REFERENCE MODEL VELOCITY : Subsystem
  MATLAB Function1 : MATLAB Function  TreatAsAtomicUnit=on
  Matrix Multiply : Product  Multiplication=Matrix(*)
  MatrixMultiply1 : Product  Multiplication=Matrix(*)
  Pseudoinverse1 : dspinverses/Pseudoinverse  wanterr=off  SimulateUsing=Interpreted execution
      settings: SourceProductBaseCode=DS
  Pseudoinverse2 : dspinverses/Pseudoinverse  wanterr=off  SimulateUsing=Interpreted execution
      settings: SourceProductBaseCode=DS
  Saturation : Saturate
  Saturation1 : Saturate
  Saturation4 : Saturate  UpperLimit=12000  LowerLimit=10
  Scope{1,7,9,11} (4 alike) : Scope
  Subsystem1 : Subsystem
  Sum{,4,6..8,11..13,16,20} (10 alike) : Sum  Inputs=|++
  Sum{1..3,17..19} (6 alike) : Sum  Inputs=|+-
  Sum15 : Sum  Inputs=|-+
  Sum21 : Sum  Inputs=|-+
  Vector Concatenate : Concatenate  NumInputs=4
  Vector Concatenate1 : Concatenate  NumInputs=4
  Vector Concatenate2 : Concatenate  NumInputs=4
  Vector Concatenate3 : Concatenate  NumInputs=3
  Motor_1_omega_input : Outport
  Motor_2_omega_input : Outport  Port=2
  Motor_3_omega_input : Outport  Port=3
  Motor_4_omega_input : Outport  Port=4
  tag scope: psi_traj=global
  wires:
  Sum13/1 -> Sum3/1  "rd_des"
  Sum4/1 -> Sum1/1  "pd_des"
  Sum2/1 -> Vector Concatenate/2
  ERROR CONTROLLER ATTITUDE/1(pd_ec) -> Sum4/2  "pd_ec"
  Sum3/1 -> Vector Concatenate/3
  ERROR CONTROLLER ATTITUDE/3(rd_ec) -> Sum13/2  "rd_ec"
  INTERNAL REFERENCE MODEL ATTITUDE/5(q_ref) -> ERROR CONTROLLER ATTITUDE/2(q_ref)  "q_ref"
  Vector Concatenate/1 -> [dv_inner], Scope1/1
  [pd_f] -> Sum1/2
  INTERNAL REFERENCE MODEL ATTITUDE/3(rd_ref) -> Sum13/1  "rd_ref"
  INTERNAL REFERENCE MODEL ATTITUDE/9(psi_ref) -> ERROR CONTROLLER ATTITUDE/6(psi_ref)  "psi_ref"
  INTERNAL REFERENCE MODEL ATTITUDE/4(p_ref) -> ERROR CONTROLLER ATTITUDE/1(p_ref)  "p_ref"
  INTERNAL REFERENCE MODEL ATTITUDE/6(r_ref) -> ERROR CONTROLLER ATTITUDE/3(r_ref)  "r_ref"
  INTERNAL REFERENCE MODEL ATTITUDE/8(theta_ref) -> ERROR CONTROLLER ATTITUDE/5(theta_ref)  "theta_ref"
  INTERNAL REFERENCE MODEL ATTITUDE/7(phi_ref) -> ERROR CONTROLLER ATTITUDE/4(phi_ref)  "phi_ref"
  ERROR CONTROLLER ATTITUDE/2(qd_ec) -> Sum11/2  "qd_ec"
  INTERNAL REFERENCE MODEL ATTITUDE/1(pd_ref) -> Sum4/1  "pd_ref"
  Sum1/1 -> Vector Concatenate/1
  Sum11/1 -> Sum2/1  "qd_des"
  [qd_f] -> Sum2/2
  INTERNAL REFERENCE MODEL ATTITUDE/2(qd_ref) -> Sum11/1  "qd_ref"
  [rd_f] -> Sum3/2
  [T_increment] -> Vector Concatenate/4
  Vector Concatenate3/1 -> Scope7/1, [dv_outer]
  Sum20/1 -> [Phi_cmd]  "phi_cmd"
  INTERNAL REFERENCE MODEL VELOCITY/5(Vy_ref) -> ERROR CONTROLLER VELOCITY/2(Vy_ref)  "Vy_ref"
  [Ax_f] -> Sum17/2
  Demux5/2 -> Sum20/1
  Sum19/1 -> Vector Concatenate3/3  "dv_z"
  8-shape trajectory/1(xd_traj) -> ?  "Vx_cmd"
  Pseudoinverse1/1 -> Scope11/1, MatrixMultiply1/1
  MatrixMultiply1/1 -> Demux5/1  "du"
  MATLAB Function1/1(B_outer) -> Scope9/1, Display1/1, Pseudoinverse1/1
  Sum21/1 -> Sum16/2  "u"
  8-shape trajectory/2(yd_traj) -> ?  "Vy_cmd"
  INTERNAL REFERENCE MODEL VELOCITY/3(Az_ref) -> Sum12/1  "Az_ref"
  Sum18/1 -> Vector Concatenate3/2  "dv_y"
  Sum6/1 -> Sum17/1
  [psi_f] -> MATLAB Function1/4(Psi)
  Sum15/1 -> Sum20/2  "u"
  Constant5/1 -> Sum15/1
  INTERNAL REFERENCE MODEL VELOCITY/2(Ay_ref) -> Sum7/1  "Ay_ref"
  Sum7/1 -> Sum18/1
  Constant8/1 -> INTERNAL REFERENCE MODEL VELOCITY/1(Vx_cmd), INTERNAL REFERENCE MODEL VELOCITY/2(Vy_cmd), INTERNAL REFERENCE MODEL VELOCITY/3(Vz_cmd)  "Vz_cmd"
  8-shape trajectory/3(psi_traj) -> [psi_traj]
  Demux5/3 -> [T_increment]  "t_incr"
  INTERNAL REFERENCE MODEL VELOCITY/1(Ax_ref) -> Sum6/1  "Ax_ref"
  Constant1/1 -> MATLAB Function1/5(m)
  ERROR CONTROLLER VELOCITY/3(Az_ec) -> Sum12/2  "Az_ec"
  INTERNAL REFERENCE MODEL VELOCITY/4(Vx_ref) -> ERROR CONTROLLER VELOCITY/1(Vx_ref)  "Vx_ref"
  ERROR CONTROLLER VELOCITY/1(Ax_ec) -> Sum6/2  "Ax_ec"
  ERROR CONTROLLER VELOCITY/2(Ay_ec) -> Sum7/2  "Ay_ec"
  Demux5/1 -> Sum16/1
  Sum12/1 -> Sum19/1
  [dv_outer] -> MatrixMultiply1/2
  Sum17/1 -> Vector Concatenate3/1  "dv_x"
  [Ay_f] -> Sum18/2
  [T_f] -> MATLAB Function1/1(T)
  INTERNAL REFERENCE MODEL VELOCITY/6(Vz_ref) -> ERROR CONTROLLER VELOCITY/3(Vz_ref)  "Vz_ref"
  [Az_f] -> Sum19/2
  Constant4/1 -> Sum21/1
  [phi_f] -> Sum15/2, MATLAB Function1/2(Phi)
  [theta_f] -> Sum21/2, MATLAB Function1/3(Theta)
  Sum16/1 -> [Theta_cmd]  "theta_cmd"
  Saturation4/1 -> Discrete Transfer Fcn/1
  Demux/4 -> Motor_4_omega_input/1
  Pseudoinverse2/1 -> Matrix Multiply/1
  Vector Concatenate2/1 -> Matrix Multiply/2
  Constant9/1 -> G2_comp/1(G2)
  Sum/1 -> Vector Concatenate2/3
  Demux1/3 -> Sum/1
  Demux1/2 -> Vector Concatenate2/2
  Constant2/1 -> G1+G2/1(G1)
  Discrete Transfer Fcn/1 -> G2_comp/2(domega)
  Constant3/1 -> G1+G2/2(G2)
  Demux/3 -> Motor_3_omega_input/1
  [omega_1_f] -> Vector Concatenate1/1
  Vector Concatenate1/1 -> G1+G2/3(omega), Sum8/2  "u"
  G2_comp/1(G2_comp) -> Sum/2  "G2_comp"
  Demux1/4 -> Vector Concatenate2/4
  Demux1/1 -> Vector Concatenate2/1
  Matrix Multiply/1 -> Saturation4/1, Sum8/1  "du"
  Demux/1 -> Motor_1_omega_input/1
  [omega_3_f] -> Vector Concatenate1/3
  Sum8/1 -> Demux/1  "u_cmd"
  Demux/2 -> Motor_2_omega_input/1
  [omega_2_f] -> Vector Concatenate1/2
  G1+G2/1(B_inner) -> Pseudoinverse2/1, Display/1  "B_inner"
  [dv_inner] -> Demux1/1  "dv_inner"
  [omega_4_f] -> Vector Concatenate1/4
  Subsystem1/1(theta_cmd) -> INTERNAL REFERENCE MODEL ATTITUDE/2(theta_cmd)  "theta_cmd"
  Saturation/1 -> INTERNAL REFERENCE MODEL ATTITUDE/1(phi_cmd)  "phi_cmd"
  Saturation1/1 -> ?  "theta_cmd"
  [Theta_cmd] -> Saturation1/1
  [Phi_cmd] -> Saturation/1
  [psi_traj] -> INTERNAL REFERENCE MODEL ATTITUDE/3(psi_cmd)

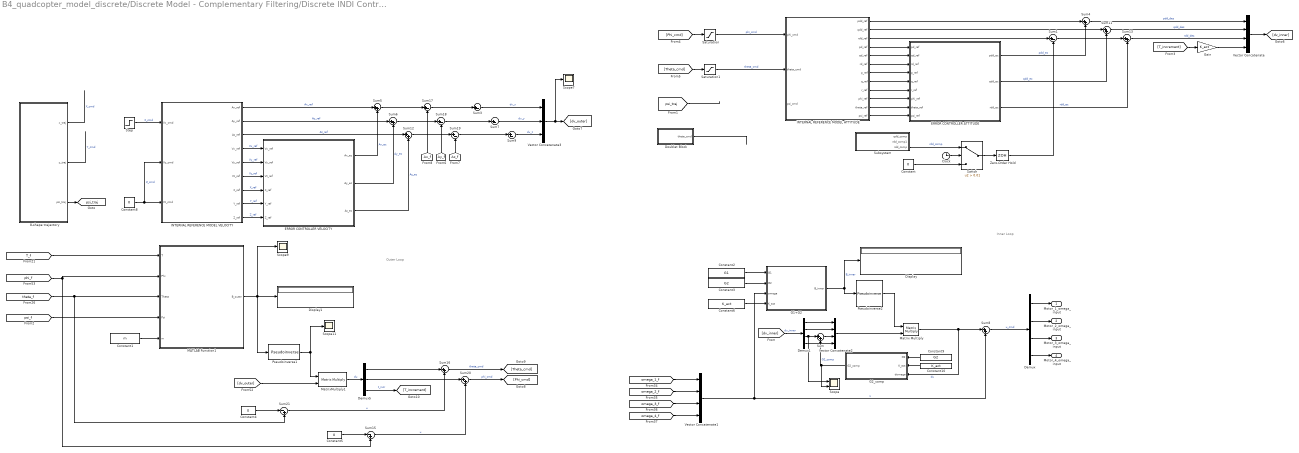
== system B4_quadcopter_model_discrete/Discrete Model - Complementary Filtering/Discrete INDI Controller Cascaded w// Actuator Compensation ==
  note: Inner Loop
  note: Outer Loop
  8-shape trajectory : Subsystem
  Clock : Clock
  Constant : Constant  Value=0  SampleTime=sampling_time
  Constant1 : Constant  Value=m  SampleTime=sampling_time
  Constant10 : Constant  Value=K_act  SampleTime=sampling_time
  Constant2 : Constant  Value=G1  SampleTime=sampling_time
  Constant3 : Constant  Value=G2  SampleTime=sampling_time
  Constant4 : Constant  Value=0
  Constant5 : Constant  Value=0
  Constant6 : Constant  Value=K_act  SampleTime=sampling_time
  Constant8 : Constant  Value=0  SampleTime=sampling_time
  Constant9 : Constant  Value=G2  SampleTime=sampling_time
  Demux : Demux
  Demux1 : Demux
  Demux5 : Demux  Outputs=3
  Display : Display
  Display1 : Display
  Doublet Block : Subsystem
  ERROR CONTROLLER ATTITUDE : Subsystem
  ERROR CONTROLLER VELOCITY : Subsystem
  G1+G2 : MATLAB Function  TreatAsAtomicUnit=on
  G2_comp : MATLAB Function  TreatAsAtomicUnit=on
  Gain : Gain  Gain=K_act
  INTERNAL REFERENCE MODEL ATTITUDE : Subsystem
  INTERNAL REFERENCE MODEL VELOCITY : Subsystem
  MATLAB Function1 : MATLAB Function  TreatAsAtomicUnit=on
  Matrix Multiply : Product  Multiplication=Matrix(*)
  MatrixMultiply1 : Product  Multiplication=Matrix(*)
  Pseudoinverse1 : dspinverses/Pseudoinverse  wanterr=off  SimulateUsing=Interpreted execution
      settings: SourceProductBaseCode=DS
  Pseudoinverse2 : dspinverses/Pseudoinverse  wanterr=off  SimulateUsing=Interpreted execution
      settings: SourceProductBaseCode=DS
  Saturation : Saturate
  Saturation1 : Saturate
  Scope : Scope  NumInputPorts=2
  Scope11 : Scope
  Scope7 : Scope
  Scope9 : Scope
  Step : Step  Time=2  After=2  SampleTime=sampling_time
  Subsystem : Subsystem
  Sum{,4..6,8,11..13,16,20} (10 alike) : Sum  Inputs=|++
  Sum{1,3,7,9,17..19} (7 alike) : Sum  Inputs=|+-
  Sum15 : Sum  Inputs=|-+
  Sum21 : Sum  Inputs=|-+
  Switch : Switch  Criteria=u2 > Threshold  Threshold=0.01
  Vector Concatenate : Concatenate  NumInputs=4
  Vector Concatenate1 : Concatenate  NumInputs=4
  Vector Concatenate2 : Concatenate  NumInputs=4
  Vector Concatenate3 : Concatenate  NumInputs=3
  Zero-Order Hold : ZeroOrderHold  SampleTime=sampling_time
  Motor_1_omega_input : Outport
  Motor_2_omega_input : Outport  Port=2
  Motor_3_omega_input : Outport  Port=3
  Motor_4_omega_input : Outport  Port=4
  tag scope: psi_traj=global
  wires:
  G1+G2/1(B_inner) -> Pseudoinverse2/1, Display/1  "B_inner"
  Vector Concatenate1/1 -> G1+G2/3(omega), Sum8/2  "u"
  Vector Concatenate/1 -> [dv_inner]
  Matrix Multiply/1 -> G2_comp/3(domega), Sum8/1  "du"
  Demux/1 -> Motor_1_omega_input/1
  [omega_4_f] -> Vector Concatenate1/4
  [omega_2_f] -> Vector Concatenate1/2
  Demux/3 -> Motor_3_omega_input/1
  Sum8/1 -> Demux/1  "u_cmd"
  Pseudoinverse2/1 -> Matrix Multiply/1
  [omega_1_f] -> Vector Concatenate1/1
  Demux/2 -> Motor_2_omega_input/1
  Demux/4 -> Motor_4_omega_input/1
  [omega_3_f] -> Vector Concatenate1/3
  INTERNAL REFERENCE MODEL VELOCITY/5(Vy_ref) -> ERROR CONTROLLER VELOCITY/2(Vy_ref)  "Vy_ref"
  Constant4/1 -> Sum21/1
  Sum16/1 -> [Theta_cmd]  "theta_cmd"
  Sum9/1 -> Vector Concatenate3/3  "dv_z"
  INTERNAL REFERENCE MODEL VELOCITY/2(Ay_ref) -> Sum6/1  "Ay_ref"
  Sum21/1 -> Sum16/2  "u"
  INTERNAL REFERENCE MODEL VELOCITY/6(Vz_ref) -> ERROR CONTROLLER VELOCITY/3(Vz_ref)  "Vz_ref"
  INTERNAL REFERENCE MODEL VELOCITY/4(Vx_ref) -> ERROR CONTROLLER VELOCITY/1(Vx_ref)  "Vx_ref"
  ERROR CONTROLLER VELOCITY/2(Ay_ec) -> Sum6/2  "Ay_ec"
  8-shape trajectory/1(x_traj) -> ?  "X_cmd"
  Sum7/1 -> Vector Concatenate3/2  "dv_y"
  ERROR CONTROLLER VELOCITY/1(Ax_ec) -> Sum5/2  "Ax_ec"
  Sum3/1 -> Vector Concatenate3/1  "dv_x"
  ERROR CONTROLLER VELOCITY/3(Az_ec) -> Sum12/2  "Az_ec"
  Sum12/1 -> Sum19/1
  Constant8/1 -> INTERNAL REFERENCE MODEL VELOCITY/2(Vy_cmd), INTERNAL REFERENCE MODEL VELOCITY/3(Vz_cmd)  "Z_cmd"
  Pseudoinverse1/1 -> Scope11/1, MatrixMultiply1/1
  Sum15/1 -> Sum20/2  "u"
  Vector Concatenate3/1 -> Scope7/1, [dv_outer]
  INTERNAL REFERENCE MODEL VELOCITY/1(Ax_ref) -> Sum5/1  "Ax_ref"
  INTERNAL REFERENCE MODEL VELOCITY/3(Az_ref) -> Sum12/1  "Az_ref"
  Sum20/1 -> [Phi_cmd]  "phi_cmd"
  [T_f] -> MATLAB Function1/1(T)
  Sum6/1 -> Sum18/1
  Constant5/1 -> Sum15/1
  [dv_outer] -> MatrixMultiply1/2
  MATLAB Function1/1(B_outer) -> Scope9/1, Display1/1, Pseudoinverse1/1
  Demux5/3 -> [T_increment]  "t_incr"
  MatrixMultiply1/1 -> Demux5/1  "du"
  8-shape trajectory/2(y_traj) -> ?  "Y_cmd"
  [T_increment] -> Gain/1
  [Ax_f] -> Sum17/2
  [Ay_f] -> Sum18/2
  [Az_f] -> Sum19/2
  [Phi_cmd] -> Saturation/1
  [theta_f] -> Sum21/2, MATLAB Function1/3(Theta)
  [phi_f] -> Sum15/2, MATLAB Function1/2(Phi)
  INTERNAL REFERENCE MODEL ATTITUDE/4(pd_ref) -> ERROR CONTROLLER ATTITUDE/1(pd_ref)
  INTERNAL REFERENCE MODEL ATTITUDE/7(p_ref) -> ERROR CONTROLLER ATTITUDE/4(p_ref)
  ERROR CONTROLLER ATTITUDE/3(rdd_ec) -> Sum13/2  "rdd_ec"
  ERROR CONTROLLER ATTITUDE/2(qdd_ec) -> Sum11/2  "qdd_ec"
  INTERNAL REFERENCE MODEL ATTITUDE/5(qd_ref) -> ERROR CONTROLLER ATTITUDE/2(qd_ref)
  INTERNAL REFERENCE MODEL ATTITUDE/11(theta_ref) -> ERROR CONTROLLER ATTITUDE/8(theta_ref)
  INTERNAL REFERENCE MODEL ATTITUDE/1(pdd_ref) -> Sum4/1
  INTERNAL REFERENCE MODEL ATTITUDE/3(rdd_ref) -> Sum1/1
  INTERNAL REFERENCE MODEL ATTITUDE/8(q_ref) -> ERROR CONTROLLER ATTITUDE/5(q_ref)
  ERROR CONTROLLER ATTITUDE/1(pdd_ec) -> Sum4/2  "pdd_ec"
  INTERNAL REFERENCE MODEL ATTITUDE/6(rd_ref) -> ERROR CONTROLLER ATTITUDE/3(rd_ref)
  INTERNAL REFERENCE MODEL ATTITUDE/10(phi_ref) -> ERROR CONTROLLER ATTITUDE/7(phi_ref)
  INTERNAL REFERENCE MODEL ATTITUDE/12(psi_ref) -> ERROR CONTROLLER ATTITUDE/9(psi_ref)
  INTERNAL REFERENCE MODEL ATTITUDE/9(r_ref) -> ERROR CONTROLLER ATTITUDE/6(r_ref)
  Sum13/1 -> Vector Concatenate/3  "rdd_des"
  Sum4/1 -> Vector Concatenate/1  "pdd_des"
  Sum11/1 -> Vector Concatenate/2  "qdd_des"
  Gain/1 -> Vector Concatenate/4
  Constant3/1 -> G1+G2/2(G2)
  Constant6/1 -> G1+G2/4(K_act)
  Constant2/1 -> G1+G2/1(G1)
  Constant9/1 -> G2_comp/1(G2)
  Constant10/1 -> G2_comp/2(K_act)
  [dv_inner] -> Demux1/1  "dv_inner"
  Sum/1 -> Vector Concatenate2/3
  Demux1/3 -> Scope/1, Sum/1
  Demux1/2 -> Vector Concatenate2/2
  Demux1/1 -> Vector Concatenate2/1
  Demux1/4 -> Vector Concatenate2/4
  Vector Concatenate2/1 -> Matrix Multiply/2
  G2_comp/1(G2_comp) -> Scope/2, Sum/2  "G2_comp"
  Sum5/1 -> Sum17/1
  Saturation1/1 -> INTERNAL REFERENCE MODEL ATTITUDE/2(theta_cmd)  "theta_cmd"
  INTERNAL REFERENCE MODEL ATTITUDE/2(qdd_ref) -> Sum11/1
  8-shape trajectory/3(psi_traj) -> [psi_traj]
  [Theta_cmd] -> Saturation1/1
  Saturation/1 -> INTERNAL REFERENCE MODEL ATTITUDE/1(phi_cmd)  "phi_cmd"
  Sum17/1 -> Sum3/1
  Sum18/1 -> Sum7/1
  Sum19/1 -> Sum9/1
  Constant1/1 -> MATLAB Function1/5(m)
  Demux5/2 -> Sum20/1
  Demux5/1 -> Sum16/1
  [psi_f] -> MATLAB Function1/4(Psi)
  [psi_traj] -> ?
  Clock/1 -> Switch/2
  Constant/1 -> Switch/3
  Zero-Order Hold/1 -> Sum1/2
  Switch/1 -> Zero-Order Hold/1
  INTERNAL REFERENCE MODEL VELOCITY/7(X_ref) -> ERROR CONTROLLER VELOCITY/4(X_ref)  "X_ref"
  INTERNAL REFERENCE MODEL VELOCITY/8(Y_ref) -> ERROR CONTROLLER VELOCITY/5(Y_ref)  "Y_ref"
  INTERNAL REFERENCE MODEL VELOCITY/9(Z_ref) -> ERROR CONTROLLER VELOCITY/6(Z_ref)  "Z_ref"
  Doublet Block/1(theta_cmd) -> ?
  Sum1/1 -> Sum13/1
  Subsystem/3(rdd_comp) -> Switch/1  "rdd_comp"
  Step/1 -> INTERNAL REFERENCE MODEL VELOCITY/1(Vx_cmd)  "X_cmd"
